simulink model "PubIfDecisionTOS_MDL"  (R2020b)
settings: configuration reference "DspaceConfig" (kept outside this file)
PostLoadFcn:
  | if any(exist('dsrtsu_mdlpostloadfcn', 'file') ~= 0), dsrtsu_mdlpostloadfcn('Execute', bdroot); end
InitFcn:
  | , if any(exist('dsmpb_private', 'file') ~= 0), dsmpb_private('dsmpb_mdlclblib', 'Init', bdroot); end,
undefined symbols (not defined in the file or in its folder): C_TOS_ACCEgoRAxletoFbumplength_m, C_TOS_ACCTargetFront_Flag, C_TOS_AEBJAPedObjDxThre_Val, C_TOS_AEBJAPedObjDyThre_Val, C_TOS_AEBJATargetSize_Val, C_TOS_AEBJAVehObjDxThre_Val, C_TOS_AEBJAVehObjDyThre_Val, C_TOS_AEBJuncPedTargetSize_Val, C_TOS_AEBLatObjDxThre_Val, C_TOS_AEBLatPedDyThre_Val, C_TOS_AEBLatTargetSize_Val, C_TOS_AEBLongTargetInEgoFront_Flag, C_TOS_axAbsGround_Parameter, C_TOS_CameraConfirmedFlag, C_TOS_CNsubjWidth, C_TOS_CurrentLaneCoreMinWidth_Val, C_TOS_CutInProb_Val_Zero, C_TOS_CutOutProb_Val_Zero, C_TOS_D2R_Val, C_TOS_DefaultValueObjectToCenterLine_dy, C_TOS_EgoCarWidth_Val, C_TOS_EgoDxRefPoint_m, C_TOS_EgoRAxletoFbumplength_m, C_TOS_HalfWidthVehicle_Con, C_TOS_HWA_CurrentLaneFlag, C_TOS_HWA_LeftLaneFlag, C_TOS_HWA_MovingDir_Vaild, C_TOS_HWA_MovState_Vaild, C_TOS_HWA_RightLaneFlag, C_TOS_LaneLineCourseErrorFront, C_TOS_LaneLineCourseErrorRear, C_TOS_MotorbikeDefaultWidth_m, C_TOS_NumberOfEffectiveTargets, C_TOS_Obj_Age_Val, C_TOS_Objdx_Constraint_Val, C_TOS_ObjectDefaultWidth_m, C_TOS_ObjInCurrentLane_Val, C_TOS_ObjInCurrentLaneValid, C_TOS_ObjInLeftLaneValid, C_TOS_ObjInRightLaneValid, C_TOS_ObjNotInCurrentLane_Val, C_TOS_ObjNotREElementType, C_TOS_ObjPredictDis_dy_ConstantVal_Zeros, C_TOS_ObjToCenterLine_ConstantVal_Zeros, C_TOS_OFMObjIDInvilad_Val, C_TOS_PIL_LatDisCons_Val_zero, C_TOS_PIL_ObjectCutInFlag_b, C_TOS_PIL_ObjectCutOutFlag_b, C_TOS_PIL_ObjLaneProb_al_Val, C_TOS_PP_ObjFusType_FC_Confirm_b, C_TOS_PP_ObjFusType_FC_FR_Confirm_b, C_TOS_PP_ObjFusType_FR_Confirm_b, C_TOS_RE_80BoolDefault_Val, C_TOS_RE_80Single181Default_Val, C_TOS_RE_80Single255Default_Val, C_TOS_RE_80Uint8Default_Val, C_TOS_RE_D2R, C_TOS_RE_D_180_Val, C_TOS_RE_InvalidObjectID_Val, C_TOS_RE_InvalidTargetChainDir_Val ... (+142)
libraries: simulink x1650, TOS_LIB x361, canfdmsglib x14
(part 5 of 69)

== system PubIfDecisionTOS_MDL/TOS_20201112/TOS_2012080320/TOS ==
  TOS_AddAttributes : Inport
  OFM_SignalVerification : Inport  Port=2
  TLJ_TargetInLaneValidityJudg : Inport  Port=3
  VIE_SignalVerification : Inport  Port=4
  PP_CenterLineCalculat : Inport  Port=5
  TOS_VCAN_SignalVerification : Inport  Port=6
  LM_SignalVerification : Inport  Port=7
  TOS_ProbInLaneCalculat : Inport  Port=8
  PP_REElementType : Inport  Port=9
  ACC : Subsystem
  AEB : Subsystem
  Bus Selector : BusSelector  OutputSignals=VIE_SignalVerification.psiDtOpt,VIE_SignalVerification.vxvRefMs
  Constant : Constant  OutDataTypeStr=boolean
  LC_LCKie_ELK : Subsystem
  OutPutPortAdaptation : Subsystem
  P0_Trajectory_V1.0 : Subsystem
  Signal Conversion{,1..12} (13 alike) : SignalConversion  OverrideOpt=off
  TOS_AEBLONOBJ : Outport  OutDataTypeStr=Bus: TOS_AEB_LONOBJ_BUS  PortDimensions=1  BusOutputAsStruct=on
  TOS_AEB_JAOBJ : Outport  Port=2  OutDataTypeStr=Bus: TOS_AEB_JAOBJ_BUS  PortDimensions=1  BusOutputAsStruct=on
  TOS_AEB_LATOBJ : Outport  Port=3  OutDataTypeStr=Bus: TOS_AEB_LATOBJ_BUS  PortDimensions=1  BusOutputAsStruct=on
  TOS_ACCP0 : Outport  Port=4  OutDataTypeStr=Bus: TOS_ACCP0_BUS  PortDimensions=1  BusOutputAsStruct=on
  TOS_ACCP1 : Outport  Port=5  OutDataTypeStr=Bus: TOS_ACCP1_BUS  PortDimensions=1  BusOutputAsStruct=on
  TOS_ACCP2 : Outport  Port=6  OutDataTypeStr=Bus: TOS_ACCP2_BUS  PortDimensions=1  BusOutputAsStruct=on
  TOS_ACCP3 : Outport  Port=7  OutDataTypeStr=Bus: TOS_ACCP3_BUS  PortDimensions=1  BusOutputAsStruct=on
  TOS_ACCP4 : Outport  Port=8  OutDataTypeStr=Bus: TOS_ACCP4_BUS  PortDimensions=1  BusOutputAsStruct=on
  TOS_ACCP5 : Outport  Port=9  OutDataTypeStr=Bus: TOS_ACCP5_BUS  PortDimensions=1  BusOutputAsStruct=on
  TOS_LC : Outport  Port=10  OutDataTypeStr=Bus: TOS_LC_BUS  PortDimensions=1  BusOutputAsStruct=on
  TOS_LCKIE : Outport  Port=11  OutDataTypeStr=Bus: TOS_LCKIE_BUS  PortDimensions=1  BusOutputAsStruct=on
  TOS_ELK : Outport  Port=12  OutDataTypeStr=Bus: TOS_ELK_BUS  PortDimensions=1  BusOutputAsStruct=on
  TEM_P0_TARGET_LINE : Outport  Port=13  OutDataTypeStr=Bus: TOS_P0_TARGET_LINE_BUS  PortDimensions=1  BusOutputAsStruct=on
  wires:
  P0_Trajectory_V1.0/1(TEM_P0_TARGET_LINE) -> Signal Conversion12/1  "TOS_TEM_P0_TARGET_LINE"
  LC_LCKie_ELK/3(TOS_ELK) -> Signal Conversion11/1  "TOS_ELK"
  LC_LCKie_ELK/2(TOS_LCKie) -> Signal Conversion10/1  "TOS_LCKIE"
  LC_LCKie_ELK/1(TOS_LC) -> Signal Conversion9/1  "TOS_LC"
  TOS_ProbInLaneCalculat/1 -> OutPutPortAdaptation/5(TOS_ProbInLaneCalculat)  "TOS_ProbInLaneCalculat"
  VIE_SignalVerification/1 -> OutPutPortAdaptation/4(VIE_SignalVerification)  "VIE_SignalVerification"
  TLJ_TargetInLaneValidityJudg/1 -> OutPutPortAdaptation/3(TLJ_TargetInLaneValidityJudg)  "TLJ_TargetInLaneValidityJudg"
  OFM_SignalVerification/1 -> OutPutPortAdaptation/2(OFM_SignalVerification)  "OFM_SignalVerification"
  TOS_AddAttributes/1 -> OutPutPortAdaptation/1(TOS_AddAttributes)  "TOS_AddAttributes"
  OutPutPortAdaptation/1(Out1) -> Bus Selector/1, LC_LCKie_ELK/1(TOSAAt_OFM_TIL_VIE), ACC/1(TOSAAt_OFM_TIL_VIE), AEB/1(TOSAAt_OFM_TIL_VIE)
  AEB/2(TOS_AEB_JAOBJ) -> Signal Conversion1/1  "TOS_AEBJuncObjInfo"
  AEB/3(TOS_AEB_LATOBJ) -> Signal Conversion2/1  "TOS_AEBLatObjInfo"
  ACC/6(TOS_ACCP5) -> Signal Conversion8/1  "TOS_ACCP5"
  ACC/5(TOS_ACCP4) -> Signal Conversion7/1  "TOS_ACCP4"
  ACC/4(TOS_ACCP3) -> Signal Conversion6/1  "TOS_ACCP3"
  ACC/3(TOS_ACCP2) -> Signal Conversion5/1  "TOS_ACCP2"
  AEB/1(TOS_AEBLONOBJ) -> Signal Conversion/1  "TOS_AEBLongObjInfo"
  ACC/2(TOS_ACCP1) -> Signal Conversion4/1  "TOS_ACCP1"
  ACC/1(TOS_ACCP0) -> Signal Conversion3/1  "TOS_ACCP0"
  PP_CenterLineCalculat/1 -> OutPutPortAdaptation/6(PP_CenterLineCalculat)  "PP_CenterLineCalculat"
  TOS_VCAN_SignalVerification/1 -> OutPutPortAdaptation/7(TOS_VCAN_SignalVerification)  "TOS_VCAN_SignalVerification"
  LM_SignalVerification/1 -> OutPutPortAdaptation/8(LM_SignalVerification)  "LM_SignalVerification"
  [TOS_ACC_P0] -> P0_Trajectory_V1.0/4(TOS_ACC_P0)
  Bus Selector/1 -> P0_Trajectory_V1.0/2(PsiDtOpt)  "<psiDtOpt>"
  Bus Selector/2 -> P0_Trajectory_V1.0/3(VxvRef_ms)  "<vxvRefMs>"
  Constant/1 -> P0_Trajectory_V1.0/1(VehStandstill)
  PP_REElementType/1 -> OutPutPortAdaptation/9(PP_REElementType)  "PP_REElementType"
  Signal Conversion/1 -> TOS_AEBLONOBJ/1
  Signal Conversion1/1 -> TOS_AEB_JAOBJ/1
  Signal Conversion2/1 -> TOS_AEB_LATOBJ/1
  Signal Conversion3/1 -> [TOS_ACC_P0], TOS_ACCP0/1
  Signal Conversion4/1 -> TOS_ACCP1/1
  Signal Conversion5/1 -> TOS_ACCP2/1
  Signal Conversion6/1 -> TOS_ACCP3/1
  Signal Conversion7/1 -> TOS_ACCP4/1
  Signal Conversion8/1 -> TOS_ACCP5/1
  Signal Conversion9/1 -> TOS_LC/1
  Signal Conversion10/1 -> TOS_LCKIE/1
  Signal Conversion11/1 -> TOS_ELK/1
  Signal Conversion12/1 -> TEM_P0_TARGET_LINE/1

== system PubIfDecisionTOS_MDL/TOS_20201112/TOS_2012080320/TOS_P0_TARGET ==
  TOS_P0_TARGET : Inport
  TOS_UpdateCnt : Inport  Port=2
  Bus Selector : BusSelector  OutputSignals=OTL_C0,OTL_C1,OTL_C2,OTL_C3,OTL_Cnt,OTL_Range,OTL_Valid
  CAN FD Pack : canfdmsglib/CAN FD Pack  CANdbFile=D:\029_HWA\05_HWA\05_详细设计文档\TOS_V3_dbc\InternalData03_ACC_AEBLog_ELK_LC_LCKie_20200927.dbc  MsgList=(none)  MsgName=TOS_P0_TARGET  ProtocolMode=CAN FD  MsgIDType=Standard (11-bit identifier)  MsgIdentifier=528  MsgLength=64  Remote=off  BRSSwitch=off  ApplyMinMax=off  SignalInfo={'{'OTL_C0','12','12','BE','unsigned','Standard','0','0.01','-16','-16','24.95';'OTL_C1','29','11','BE','unsigned','Standard','0','0.0009','-0.9','-0.9','0.9423';'OTL_C2','44','12','BE','unsigned','Standard','0','5e-06','-0.01','-0.01','0.010475';'OTL_C3','56','16','BE','unsigned','Standard','0','1e-08','-0.00033','-0.00033','0.00032535';'OTL_Cnt','64','8','BE','unsigned','Standard','0','1','0','0','255';'OTL_Range','85','11','BE','unsigned','Standard','0','0.1','0','0','204.7';'OTL_Valid','10','2','BE','unsigned','Standard','0','1','0','0','3'}
      settings: SourceProductBaseCode=VN  DataFormat=CANdb specified signals
  TOS_P0_TARGET_msg : Outport
  wires:
  CAN FD Pack/1 -> TOS_P0_TARGET_msg/1
  TOS_P0_TARGET/1 -> Bus Selector/1
  Bus Selector/1 -> CAN FD Pack/1  "<OTL_C0>"
  Bus Selector/2 -> CAN FD Pack/2  "<OTL_C1>"
  Bus Selector/3 -> CAN FD Pack/3  "<OTL_C2>"
  Bus Selector/4 -> CAN FD Pack/4  "<OTL_C3>"
  Bus Selector/5 -> CAN FD Pack/5  "<OTL_Cnt>"
  Bus Selector/6 -> CAN FD Pack/6  "<OTL_Range>"
  Bus Selector/7 -> CAN FD Pack/7  "<OTL_Valid>"
  TOS_UpdateCnt/1 -> CAN FD Pack/8

== system PubIfDecisionTOS_MDL/TOS_20201112/TOS_2012080320/PIL_1029/BoundaryCalculat ==
  OFM_SignalVerification : Inport
  TOS_AddAttributes : Inport  Port=2
  PP_Same_CenterLine : Inport  Port=3
  PP_Left_CenterLine : Inport  Port=4
  PP_Right_CenterLine : Inport  Port=5
  PP_CenterLineCalculat : Inport  Port=6
  Bus Creator1 : BusCreator  Inputs=12
  Bus Creator3 : BusCreator  Inputs=6
  Bus Creator5 : BusCreator  Inputs=3
  Bus Selector1 : BusSelector  OutputSignals=OFM_SignalVerification,TOS_AddAttributes,PP_CenterLineCalculat
  Bus Selector4 : BusSelector  OutputSignals=OFM_SignalVerification,PP_Left_CenterLine,PP_Same_CenterLine,PP_Right_CenterLine
  Lane_BoundaryCalculat : Subsystem
  ObjectToCenterLine_dyc : Subsystem
  PIL_Lane_BoundaryCalculat : Outport
  PIL_ObjectToCenterLine_dyc : Outport  Port=2
  wires:
  Lane_BoundaryCalculat/12(RightLane_BasicLaneWidth_ObserVale) -> Bus Creator1/12  "RightLane_BasicLaneWidth_ObserVale"
  Lane_BoundaryCalculat/11(LeftLane_BasicLaneWidth_ObserVale) -> Bus Creator1/11  "LeftLane_BasicLaneWidth_ObserVale"
  Lane_BoundaryCalculat/10(SameLane_BasicLaneWidth_ObserVale) -> Bus Creator1/10  "SameLane_BasicLaneWidth_ObserVale"
  Bus Creator5/1 -> PIL_ObjectToCenterLine_dyc/1  "PIL_ObjectToCenterLine_dyc"
  Lane_BoundaryCalculat/9(RightLane_EdgeRight_Boundary) -> Bus Creator1/9  "RightLane_EdgeRight_Boundary"
  Lane_BoundaryCalculat/8(RightLane_EdgeLeft_Boundary) -> Bus Creator1/8  "RightLane_EdgeLeft_Boundary"
  Lane_BoundaryCalculat/7(RightLane_CoreArea_Boundary) -> Bus Creator1/7  "RightLane_CoreArea_Boundary"
  Lane_BoundaryCalculat/6(LeftLane_EdgeRight_Boundary) -> Bus Creator1/6  "LeftLane_EdgeRight_Boundary"
  Lane_BoundaryCalculat/5(LeftLane_EdgeLeft_Boundary) -> Bus Creator1/5  "LeftLane_EdgeLeft_Boundary"
  Lane_BoundaryCalculat/4(LeftLane_CoreArea_Boundary) -> Bus Creator1/4  "LeftLane_CoreArea_Boundary"
  Lane_BoundaryCalculat/3(SameLane_EdgeRight_Boundary) -> Bus Creator1/3  "SameLane_EdgeRight_Boundary"
  Lane_BoundaryCalculat/2(SameLane_EdgeLeft_Boundary) -> Bus Creator1/2  "SameLane_EdgeLeft_Boundary"
  Lane_BoundaryCalculat/1(SameLane_CoreArea_Boundary) -> Bus Creator1/1  "SameLane_CoreArea_Boundary"
  ObjectToCenterLine_dyc/3(PIL_RightCenterLine_dyc_Filt) -> Bus Creator5/3  "PIL_RightCenterLine_dyc"
  ObjectToCenterLine_dyc/2(PIL_SameCenterLine_dyc_Filt) -> Bus Creator5/2  "PIL_SameCenterLine_dyc"
  ObjectToCenterLine_dyc/1(PIL_LeftCenterLine_dyc_Filt) -> Bus Creator5/1  "PIL_LeftCenterLine_dyc"
  Bus Selector4/1 -> ObjectToCenterLine_dyc/1(OFM_SignalVerification)  "<OFM_SignalVerification>"
  Bus Selector4/4 -> ObjectToCenterLine_dyc/4(Right_CenterLine)  "<PP_Right_CenterLine>"
  Bus Selector4/3 -> ObjectToCenterLine_dyc/3(Same_CenterLine)  "<PP_Same_CenterLine>"
  Bus Selector4/2 -> ObjectToCenterLine_dyc/2(Left_CenterLine)  "<PP_Left_CenterLine>"
  Bus Selector1/3 -> Lane_BoundaryCalculat/3(PP_CenterLineCalculat)  "<PP_CenterLineCalculat>"
  PP_CenterLineCalculat/1 -> Bus Creator3/6  "PP_CenterLineCalculat"
  Bus Creator1/1 -> PIL_Lane_BoundaryCalculat/1  "PIL_Lane_BoundaryCalculat"
  Bus Selector1/2 -> Lane_BoundaryCalculat/2(TOS_AddAttributes)  "<TOS_AddAttributes>"
  Bus Selector1/1 -> Lane_BoundaryCalculat/1(OFM_SignalVerification)  "<OFM_SignalVerification>"
  Bus Creator3/1 -> Bus Selector1/1, Bus Selector4/1
  PP_Right_CenterLine/1 -> Bus Creator3/5  "PP_Right_CenterLine"
  PP_Left_CenterLine/1 -> Bus Creator3/4  "PP_Left_CenterLine"
  PP_Same_CenterLine/1 -> Bus Creator3/3  "PP_Same_CenterLine"
  OFM_SignalVerification/1 -> Bus Creator3/1  "OFM_SignalVerification"
  TOS_AddAttributes/1 -> Bus Creator3/2  "TOS_AddAttributes"

== system PubIfDecisionTOS_MDL/TOS_20201112/TOS_2012080320/PIL_1029/ObjCutInOut_Prob ==
  PIL_ObjectToCenterLine_dy_Filt : Inport
  OFM_SignalVerification : Inport  Port=2
  TOS_AddAttributes : Inport  Port=3
  LaneWidth : Inport  Port=4
  Bus Creator : BusCreator  Inputs=4
  Bus Selector1 : BusSelector  OutputSignals=TOS_AddAttributes.PP_ObjectToCenterLine_dy,TOS_AddAttributes.PP_ObjectToCenterLine_vyc,LaneWidth.TOS_PP_CurrentLaneWidth
  Bus Selector2 : BusSelector  OutputSignals=PIL_ObjectToCenterLine_dy_Filt
  Bus Selector3 : BusSelector  OutputSignals=OFM_SignalVerification.TOS_OFMObjValid_Flag,OFM_SignalVerification.Object_Width,OFM_SignalVerification.Object_DX,OFM_SignalVerification.Object_DY,OFM_SignalVerification.Object_Age,OFM_SignalVerification.Object_Type,OFM_SignalVerification.Object_MovingState
  Bus Selector4 : BusSelector  OutputSignals=OFM_SignalVerification.TOS_OFMObjValid_Flag,OFM_SignalVerification.Object_Width,OFM_SignalVerification.Object_DX,OFM_SignalVerification.Object_DY,OFM_SignalVerification.Object_Age,OFM_SignalVerification.Object_Type,OFM_SignalVerification.Object_MovingState,OFM_SignalVerification.Object_VY,OFM_SignalVerification.Object_Std_DY
  Bus Selector5 : BusSelector  OutputSignals=TOS_AddAttributes.PP_ObjectToCenterLine_dy,TOS_AddAttributes.PP_ObjectToCenterLine_vyc
  Bus Selector6 : BusSelector  OutputSignals=PIL_ObjectToCenterLine_dy_Filt
  ObjectCutIn : Subsystem
  ObjectCutOut : Subsystem
  PIL_ObjectCutInPro_Filt : Outport
  PIL_ObjectCutIn_Flag : Outport  Port=2
  PIL_ObjectCutOutPro : Outport  Port=3
  PIL_ObjectCutOutFlag : Outport  Port=4
  wires:
  LaneWidth/1 -> Bus Creator/4  "LaneWidth"
  Bus Selector6/1 -> ObjectCutOut/12(PIL_ObjectToCenterLine_dy_Filt)  "<PIL_ObjectToCenterLine_dy_Filt>"
  Bus Selector5/2 -> ObjectCutOut/11(PP_ObjectToCenterLine_vyc)  "<PP_ObjectToCenterLine_vyc>"
  Bus Selector5/1 -> ObjectCutOut/10(PP_ObjectToCenterLine_dy)  "<PP_ObjectToCenterLine_dy>"
  Bus Selector2/1 -> ObjectCutIn/11(PIL_ObjectToCenterLine_dy_Filt)  "<PIL_ObjectToCenterLine_dy_Filt>"
  Bus Selector1/3 -> ObjectCutIn/10(PP_CurrentLaneWidth)  "<TOS_PP_CurrentLaneWidth>"
  Bus Selector1/2 -> ObjectCutIn/9(PP_ObjectToCenterLine_vyc)  "<PP_ObjectToCenterLine_vyc>"
  Bus Selector1/1 -> ObjectCutIn/8(PP_ObjectToCenterLine_dy)  "<PP_ObjectToCenterLine_dy>"
  PIL_ObjectToCenterLine_dy_Filt/1 -> Bus Creator/3  "PIL_ObjectToCenterLine_dy_Filt"
  TOS_AddAttributes/1 -> Bus Creator/2  "TOS_AddAttributes"
  OFM_SignalVerification/1 -> Bus Creator/1  "OFM_SignalVerification"
  Bus Creator/1 -> Bus Selector3/1, Bus Selector6/1, Bus Selector5/1, Bus Selector4/1, Bus Selector2/1, Bus Selector1/1
  Bus Selector4/1 -> ObjectCutOut/1(TOS_OFMObjValid_Flag)  "<TOS_OFMObjValid_Flag>"
  Bus Selector4/2 -> ObjectCutOut/2(Object_Width)  "<Object_Width>"
  Bus Selector4/3 -> ObjectCutOut/3(Object_DX)  "<Object_DX>"
  Bus Selector4/4 -> ObjectCutOut/4(Object_DY)  "<Object_DY>"
  Bus Selector4/5 -> ObjectCutOut/5(Object_Age)  "<Object_Age>"
  Bus Selector4/6 -> ObjectCutOut/6(Object_Type)  "<Object_Type>"
  Bus Selector4/7 -> ObjectCutOut/7(Object_MovingState)  "<Object_MovingState>"
  Bus Selector4/8 -> ObjectCutOut/8(Object_VY)  "<Object_VY>"
  Bus Selector4/9 -> ObjectCutOut/9(Object_Std_DY)  "<Object_Std_DY>"
  ObjectCutOut/2(TOS_PIL_ObjectCutOut_Flag) -> PIL_ObjectCutOutFlag/1
  ObjectCutOut/1(TOS_PIL_ObjectCutOutPro_Filt) -> PIL_ObjectCutOutPro/1
  Bus Selector3/1 -> ObjectCutIn/1(TOS_OFMObjValid_Flag)  "<TOS_OFMObjValid_Flag>"
  Bus Selector3/2 -> ObjectCutIn/2(Object_Width)  "<Object_Width>"
  Bus Selector3/3 -> ObjectCutIn/3(Object_DX)  "<Object_DX>"
  Bus Selector3/4 -> ObjectCutIn/4(Object_DY)  "<Object_DY>"
  Bus Selector3/5 -> ObjectCutIn/5(Object_Age)  "<Object_Age>"
  Bus Selector3/6 -> ObjectCutIn/6(Object_Type)  "<Object_Type>"
  Bus Selector3/7 -> ObjectCutIn/7(Object_MovingState)  "<Object_MovingState>"
  ObjectCutIn/1(TOS_PIL_ObjectCutInPro_Filt) -> PIL_ObjectCutInPro_Filt/1
  ObjectCutIn/2(TOS_PIL_ObjectCutIn_Flag) -> PIL_ObjectCutIn_Flag/1

== system PubIfDecisionTOS_MDL/TOS_20201112/TOS_2012080320/PIL_1029/OverlapRatio_Calculate ==
  TOS_OFMObjValid_Flag : Inport  Partition=on  PartitionDimension=1  PartitionWidth=1  PartitionOffset=0
  ObjectWidth : Inport  Port=2  Partition=on  PartitionDimension=1  PartitionWidth=1  PartitionOffset=0
  ObjectTypeCameraConfirmed : Inport  Port=3  Partition=on  PartitionDimension=1  PartitionWidth=1  PartitionOffset=0
  object_MovingState : Inport  Port=4  Partition=on  PartitionDimension=1  PartitionWidth=1  PartitionOffset=0
  Object_Type : Inport  Port=5  Partition=on  PartitionDimension=1  PartitionWidth=1  PartitionOffset=0
  dyEgo2Center : Inport  Port=6
  dyObject2Center : Inport  Port=7  Partition=on  PartitionDimension=1  PartitionWidth=1  PartitionOffset=0
  Compare To Constant : simulink/Logic and Bit Operations/Compare To Constant  relop===  const=C_TOS_OFMObjIDInvilad_Val  OutDataTypeStr=boolean
      settings: AttributesFormatString=C_TOS_OFMObjIDInvilad_Val = 0
  For Each : ForEach  DisableCoverage=on
  If : If  IfExpression=u1 ~= 0
  Merge : Merge
  OverlapCalculation_Default : Subsystem  TreatAsAtomicUnit=on
  PIL_OverlapCalculation : Subsystem  TreatAsAtomicUnit=on
  PIL_OverlapRatio : Outport  OutDataTypeStr=single  ConcatenationDimension=1
  wires:
  dyObject2Center/1 -> PIL_OverlapCalculation/6(dyObject2Center)
  dyEgo2Center/1 -> PIL_OverlapCalculation/5(dyEgo2Center)
  object_MovingState/1 -> PIL_OverlapCalculation/3(object_MovingState)
  ObjectTypeCameraConfirmed/1 -> PIL_OverlapCalculation/2(ObjectTypeCameraConfirmed)
  ObjectWidth/1 -> PIL_OverlapCalculation/1(ObjectWidth)
  OverlapCalculation_Default/1(PIL_overlapRatio) -> Merge/1
  Merge/1 -> PIL_OverlapRatio/1
  If/1 -> OverlapCalculation_Default/Action
  Compare To Constant/1 -> If/1
  TOS_OFMObjValid_Flag/1 -> Compare To Constant/1
  PIL_OverlapCalculation/1(overlapRatio) -> Merge/2
  If/2 -> PIL_OverlapCalculation/Action
  Object_Type/1 -> PIL_OverlapCalculation/4(Object_Type)

== system PubIfDecisionTOS_MDL/TOS_20201112/TOS_2012080320/PIL_1029/PIL_ObjectToCenterLine_dy_Filt ==
  note: fun: 目标到本车道中心线距离滤波
  ObjectToCenterLine_dy : Inport
  TOS_OFMObjValid_Flag : Inport  Port=2
  Object_ID : Inport  Port=3  OutDataTypeStr=uint8
  Object_Age : Inport  Port=4
  PIL_ObjectToCenterLine_dy : Subsystem
  Unit Delay : UnitDelay  InitialCondition=zeros(80,1)  SampleTime=-1  HasFrameUpgradeWarning=on
      settings: AttributesFormatString=initVal = zeros(80,1)
  Unit Delay1 : UnitDelay  InitialCondition=ones(80,1)*255  SampleTime=-1  HasFrameUpgradeWarning=on
      settings: AttributesFormatString=initVal = ones(80,1)*255
  PIL_ObjectToCenterLine_dy_Filt : Outport  OutDataTypeStr=single
  wires:
  TOS_OFMObjValid_Flag/1 -> PIL_ObjectToCenterLine_dy/4(TOS_OFMObjValid_Flag)
  Object_Age/1 -> PIL_ObjectToCenterLine_dy/6(Object_Age)
  ObjectToCenterLine_dy/1 -> PIL_ObjectToCenterLine_dy/3(ObjectToCenterLine_dy)
  PIL_ObjectToCenterLine_dy/2(ObjectToCenterLine_dy_Filt) -> PIL_ObjectToCenterLine_dy_Filt/1, Unit Delay1/1  "TOS_PIL_ObjectToCenterLine_dy_Filt"
  Unit Delay1/1 -> PIL_ObjectToCenterLine_dy/2(ObjectToCenterLine_dy_Filt_K1)
  Object_ID/1 -> PIL_ObjectToCenterLine_dy/5(Object_ID)
  PIL_ObjectToCenterLine_dy/1(Obj_ID) -> Unit Delay/1
  Unit Delay/1 -> PIL_ObjectToCenterLine_dy/1(ObjectID_Filt_K1)

== system PubIfDecisionTOS_MDL/TOS_20201112/TOS_2012080320/PIL_1029/ProbCalculat ==
  CurrentLane_LeftRightLine : Inport
  OFM_SignalVerification : Inport  Port=2
  TOS_AddAttributes : Inport  Port=3
  LM_SignalVerification : Inport  Port=4
  PIL_Lane_BoundaryCalculat : Inport  Port=5
  PIL_ObjectToCenterLine_dyc : Inport  Port=6
  Bus Creator : BusCreator  Inputs=6
  Bus Selector : BusSelector  OutputSignals=OFM_SignalVerification,PIL_Lane_BoundaryCalculat,PIL_ObjectToCenterLine_dyc,LM_SignalVerification
  ProbCalculat : Subsystem
  ProbFilt : Subsystem
  PIL_ObjinEgoLaneProb_Filt : Outport  OutDataTypeStr=single
  PIL_ObjinLeftLaneProb_Filt : Outport  Port=2  OutDataTypeStr=single
  PIL_ObjinRightLaneProb_Filt : Outport  Port=3  OutDataTypeStr=single
  "PIL_ObjLaneProb_all " : Outport  Port=4
  PIL_EgoVehicleProFilt : Outport  Port=5
  wires:
  ProbFilt/1(PIL_ObjinEgoLaneProb_Filt) -> [TOS_PIL_SameLanePro_Filt], PIL_ObjinEgoLaneProb_Filt/1
  ProbFilt/3(PIL_ObjinRightLaneProb_Filt) -> [PIL_RightLaneProb_Filt], PIL_ObjinRightLaneProb_Filt/1
  ProbFilt/2(PIL_ObjinLeftLaneProb_Filt) -> [PIL_LeftLaneProb_Filt], PIL_ObjinLeftLaneProb_Filt/1
  Bus Creator/1 -> [OFM_InPutSig], Bus Selector/1
  ProbCalculat/3(PIL_RightLaneProb) -> ProbFilt/4(PIL_ObjinRightLaneProb), [TOS_PIL_RightLaneProb]
  ProbCalculat/2(PIL_LeftLaneProb) -> ProbFilt/3(PIL_ObjinLeftLaneProb), [PIL_LeftLaneProb]
  Bus Selector/3 -> ProbCalculat/3(PIL_ObjectToCenterLine_dyc)  "<PIL_ObjectToCenterLine_dyc>"
  TOS_AddAttributes/1 -> Bus Creator/3  "TOS_AddAttributes"
  CurrentLane_LeftRightLine/1 -> Bus Creator/1  "CurrentLane_LeftRightLine"
  Bus Selector/2 -> ProbCalculat/2(CurrentLane_Boundary)  "<PIL_Lane_BoundaryCalculat>"
  Bus Selector/1 -> ProbCalculat/1(OFM_SignalVerification)  "<OFM_SignalVerification>"
  PIL_ObjectToCenterLine_dyc/1 -> Bus Creator/6  "PIL_ObjectToCenterLine_dyc"
  PIL_Lane_BoundaryCalculat/1 -> Bus Creator/5  "PIL_Lane_BoundaryCalculat"
  OFM_SignalVerification/1 -> Bus Creator/2  "OFM_SignalVerification"
  ProbCalculat/1(PIL_EgoLaneProb) -> ProbFilt/2(PIL_ObjinEgoLaneProb), [PIL_CurrentLaneProb]
  LM_SignalVerification/1 -> Bus Creator/4  "LM_SignalVerification"
  Bus Selector/4 -> ProbCalculat/4(LM_SignalVerification)  "<LM_SignalVerification>"
  ProbCalculat/5(PIL_EgoVehicleProFilt) -> [PIL_EgoVehicleProFilt], PIL_EgoVehicleProFilt/1
  ProbCalculat/4("PIL_ObjLaneProb_all ") -> "PIL_ObjLaneProb_all "/1
  [OFM_InPutSig] -> ProbFilt/1(OFM_InPutSig)

== system PubIfDecisionTOS_MDL/TOS_20201112/TOS_2012080320/PP1128/AAT-AdditionalAttributes ==
  LM_SignalVerification : Inport
  OFM_Info : Inport  Port=2
  VIE_SignalVerification : Inport  Port=3
  Bus Creator : BusCreator  Inputs=3
  Bus Creator1 : BusCreator  Inputs=14  OutDataTypeStr=Bus: TOS_AddAttributes_BUS  NonVirtualBus=on
      settings: InheritFromInputs=off
  Bus Creator3 : BusCreator  Inputs=4
  Bus Selector : BusSelector  OutputSignals=OFM_SignalVerification.Object_MovingState,OFM_SignalVerification.Object_Orientation,OFM_SignalVerification.Object_AX,VIE_SignalVerification.axvRefMs2,OFM_SignalVerification.Object_MovingState,OFM_SignalVerification.Object_Fus_Type,OFM_SignalVerification.Object_DX,OFM_SignalVerification.TOS_OFMObjValid_Flag
  Bus Selector1 : BusSelector  OutputSignals=OFM_SignalVerification,LM_SignalVerification,VIE_SignalVerification
  Bus Selector3 : BusSelector  OutputSignals=OFM_SignalVerification.Object_DX,OFM_SignalVerification.Object_DY,OFM_SignalVerification.Object_ID,OFM_SignalVerification.TOS_OFMObjValid_Flag
  Bus Selector5 : BusSelector  OutputSignals=OFM_SignalVerification,LM_SignalVerification,VIE_SignalVerification.vxvRefMs
  Bus Selector6 : BusSelector  OutputSignals=OFM_SignalVerification,LM_SignalVerification
  PP_CenterLine_Calculat : Subsystem
  PP_ObjFirstDxDyDetermineSignalProcessing : Subsystem
  PP_ObjectToCenterLine_dy : Subsystem
  PP_SignalProcessing : Subsystem
  RoadEdge : Subsystem
  TAP_TargetPreprocessing : Subsystem
  TOS_AddAttributes : Outport
  PP_CenterLineCalculat : Outport  Port=2
  OFM_SignalVerification : Outport  Port=3
  PP_REElementType : Outport  Port=4
  wires:
  LM_SignalVerification/1 -> Bus Creator/3  "LM_SignalVerification"
  OFM_Info/1 -> TAP_TargetPreprocessing/1(OFM_Info)  "OFM_SignalVerification"
  Bus Selector5/1 -> PP_ObjectToCenterLine_dy/1("OFM_SignalVerification ")  "<OFM_SignalVerification>"
  Bus Selector5/2 -> PP_ObjectToCenterLine_dy/2(LM_SignalVerification)  "<LM_SignalVerification>"
  PP_ObjectToCenterLine_dy/2(PP_ObjectToCenterLine_dy) -> Bus Creator1/11  "TOS_PP_ObjectToCenterLine_dy"
  VIE_SignalVerification/1 -> Bus Creator/2  "VIE_SignalVerification"
  Bus Creator1/1 -> TOS_AddAttributes/1  "TOS_PP_AddAttributes_bus"
  Bus Selector3/1 -> PP_ObjFirstDxDyDetermineSignalProcessing/1(Object_DX)  "<Object_DX>"
  Bus Selector3/2 -> PP_ObjFirstDxDyDetermineSignalProcessing/2(Object_DY)  "<Object_DY>"
  Bus Selector3/3 -> PP_ObjFirstDxDyDetermineSignalProcessing/3(Object_ID)  "<Object_ID>"
  PP_ObjectToCenterLine_dy/1(PP_EgoVehCenterLine_dy) -> Bus Creator1/10  "TOS_PP_EgoVehCenterLine_dy"
  PP_ObjFirstDxDyDetermineSignalProcessing/1(PP_ObjFirstDetect_Dx) -> Bus Creator1/13  "PP_ObjFirstDetect_Dx"
  PP_ObjFirstDxDyDetermineSignalProcessing/2(PP_ObjFirstDetect_Dy) -> Bus Creator1/14  "PP_ObjFirstDetect_Dy"
  PP_ObjectToCenterLine_dy/3(PP_ObjectToCenterLine_Vyc) -> Bus Creator1/12  "PP_ObjectToCenterLine_vyc"
  Bus Selector5/3 -> PP_ObjectToCenterLine_dy/3(vxvRefMs)  "<vxvRefMs>"
  Bus Selector/1 -> PP_SignalProcessing/1(Object_MovingState)  "<Object_MovingState>"
  Bus Selector/2 -> PP_SignalProcessing/2(Object_Orientation)  "<Object_Orientation>"
  Bus Selector/3 -> PP_SignalProcessing/3(Object_AX)  "<Object_AX>"
  Bus Selector/4 -> PP_SignalProcessing/4(axvRefMs2)  "<axvRefMs2>"
  Bus Selector/5 -> PP_SignalProcessing/5(Object_MovingState1)  "<Object_MovingState>"
  Bus Selector/6 -> PP_SignalProcessing/6(Object_Fus_Type)  "<Object_Fus_Type>"
  Bus Selector/7 -> PP_SignalProcessing/7(Object_DX)  "<Object_DX>"
  PP_SignalProcessing/1(PP_MovingStateSignalProcessing) -> Bus Creator1/1  "PP_MovingStateSignalProcessing"
  PP_SignalProcessing/4(PP_axAbsGround) -> Bus Creator1/4  "PP_axAbsGround"
  PP_SignalProcessing/5(PP_CamareConfirmSignalProcessing) -> Bus Creator1/5  "PP_CamareConfirmSignalProcessing"
  PP_SignalProcessing/6(PP_ObjToEgoCarFrontbump) -> Bus Creator1/6  "PP_ObjToEgoCarFrontbump"
  PP_CenterLine_Calculat/4(PP_LaneWidth) -> Bus Creator3/4
  Bus Creator3/1 -> PP_CenterLineCalculat/1  "PP_CenterLineCalculat"
  PP_CenterLine_Calculat/3(PP_RightLane_CenterLine) -> Bus Creator3/3
  PP_CenterLine_Calculat/2(PP_LeftLane_CenterLine) -> Bus Creator3/2
  Bus Selector6/2 -> PP_CenterLine_Calculat/2(LM_SignalVerification)  "<LM_SignalVerification>"
  PP_CenterLine_Calculat/1(PP_EgoLane_CenterLine) -> Bus Creator3/1
  Bus Selector/8 -> PP_SignalProcessing/8(TOS_OFMObjValid_Flag)  "<TOS_OFMObjValid_Flag>"
  PP_SignalProcessing/3(PP_ObjMovingDirSignalProcessing) -> Bus Creator1/3  "PP_ObjMovingDirSignalProcessing"
  TAP_TargetPreprocessing/1(OFM_SignalVerification) -> OFM_SignalVerification/1, Bus Creator/1  "OFM_SignalVerification"
  Bus Selector3/4 -> PP_ObjFirstDxDyDetermineSignalProcessing/4(TOS_OFMObjValid_Flag)  "<TOS_OFMObjValid_Flag>"
  PP_SignalProcessing/7(PP_ObjFusType_FC_FR_Confirm) -> Bus Creator1/7  "PP_ObjFusType_FC_FR_Confirm"
  PP_SignalProcessing/8(PP_ObjFusType_FR_Confirm) -> Bus Creator1/8  "PP_ObjFusType_FR_Confirm"
  PP_SignalProcessing/9(PP_ObjFusType_FC_Confirm) -> Bus Creator1/9  "PP_ObjFusType_FC_Confirm"
  Bus Selector6/1 -> PP_CenterLine_Calculat/1(OFM_SignalVerification)  "<OFM_SignalVerification>"
  PP_SignalProcessing/2(PP_MovingState_AEB_SignalProcessing) -> Bus Creator1/2  "PP_MovingState_AEB_SignalProcessing"
  Bus Selector1/3 -> RoadEdge/3(VIE_SignalVerification)  "<VIE_SignalVerification>"
  Bus Selector1/1 -> RoadEdge/1(OFM_SignalVerification)  "<OFM_SignalVerification>"
  RoadEdge/1(RE_EdgeElementType) -> PP_REElementType/1
  Bus Selector1/2 -> RoadEdge/2(LM_SignalVerification)  "<LM_SignalVerification>"
  Bus Creator/1 -> Bus Selector/1, Bus Selector1/1, Bus Selector6/1, Bus Selector3/1, Bus Selector5/1

== system PubIfDecisionTOS_MDL/TOS_20201112/TOS_2012080320/PP1128/ISV_InputSignalVerification ==
  OFMInfo : Inport
  vxvRefMs : Inport  Port=2
  psiDtOpt : Inport  Port=3  Interpolate=off
  kapTraj : Inport  Port=4
  axvRefMs2 : Inport  Port=5
  TOS_VCAN_CSA : Inport  Port=6  BusOutputAsStruct=on
  LM_LINE_LL : Inport  Port=7  BusOutputAsStruct=on
  LM_LINE_LR : Inport  Port=8  BusOutputAsStruct=on
  LM_LINE_RL : Inport  Port=9  BusOutputAsStruct=on
  LM_LINE_RR : Inport  Port=10  BusOutputAsStruct=on
  LM_SpecialRoadType : Inport  Port=11  OutDataTypeStr=uint8  PortDimensions=1  BusOutputAsStruct=on
  LM_RoadNumChgType : Inport  Port=12  OutDataTypeStr=uint8  PortDimensions=1  BusOutputAsStruct=on
  LM_DrivInWLType : Inport  Port=13  OutDataTypeStr=uint8  PortDimensions=1  BusOutputAsStruct=on
  LM_SignalVerif : Subsystem
  OFM_SignalVerif : Subsystem
  VIE_SignalVerif : Subsystem
  LM_SignalVerification : Outport
  OFM_SignalVerification : Outport  Port=2
  VIE_SignalVerification : Outport  Port=3
  TOS_VCAN_SignalVerification : Outport  Port=4
  wires:
  TOS_VCAN_CSA/1 -> TOS_VCAN_SignalVerification/1
  OFMInfo/1 -> OFM_SignalVerif/1(OFMInfo)  "OFMInfo"
  OFM_SignalVerif/1(OFM_SignalVerification) -> OFM_SignalVerification/1
  vxvRefMs/1 -> VIE_SignalVerif/1(vxvRefMs)
  psiDtOpt/1 -> VIE_SignalVerif/2(psiDtOpt)
  kapTraj/1 -> VIE_SignalVerif/3(kapTraj)
  axvRefMs2/1 -> VIE_SignalVerif/4(axvRefMs2)
  VIE_SignalVerif/1(VIE_SignalVerification) -> VIE_SignalVerification/1
  LM_LINE_LL/1 -> LM_SignalVerif/1(LM_LINE_LL)
  LM_LINE_LR/1 -> LM_SignalVerif/2(LM_LINE_LR)
  LM_LINE_RL/1 -> LM_SignalVerif/3(LM_LINE_RL)
  LM_LINE_RR/1 -> LM_SignalVerif/4(LM_LINE_RR)
  LM_SpecialRoadType/1 -> LM_SignalVerif/5(LM_SpecialRoadType)
  LM_RoadNumChgType/1 -> LM_SignalVerif/6(LM_RoadNumChgType)
  LM_DrivInWLType/1 -> LM_SignalVerif/7(LM_DrivInWLType)
  LM_SignalVerif/1(LM_SignalVerification) -> LM_SignalVerification/1

== system PubIfDecisionTOS_MDL/TOS_20201112/TOS_2012080320/Subsystem/For Each Subsystem ==
  In1 : Inport  Partition=on  PartitionDimension=1  PartitionWidth=1  PartitionOffset=0
  Bus Selector2 : BusSelector  OutputSignals=FusionType,ObjectID,ObjectMovingOrientation,ObjectMovingState,ObjectType,dx,dy
  For Each : ForEach  DisableCoverage=on
  FusionType : Outport  ConcatenationDimension=1
  ObjectID : Outport  Port=2  ConcatenationDimension=1
  ObjectMovingOrientation : Outport  Port=3  ConcatenationDimension=1
  ObjectMovingState : Outport  Port=4  ConcatenationDimension=1
  ObjectType : Outport  Port=5  ConcatenationDimension=1
  dx : Outport  Port=6  ConcatenationDimension=1
  dy : Outport  Port=7  ConcatenationDimension=1
  wires:
  In1/1 -> Bus Selector2/1
  Bus Selector2/1 -> FusionType/1  "<FusionType>"
  Bus Selector2/2 -> ObjectID/1  "<ObjectID>"
  Bus Selector2/3 -> ObjectMovingOrientation/1  "<ObjectMovingOrientation>"
  Bus Selector2/4 -> ObjectMovingState/1  "<ObjectMovingState>"
  Bus Selector2/5 -> ObjectType/1  "<ObjectType>"
  Bus Selector2/6 -> dx/1  "<dx>"
  Bus Selector2/7 -> dy/1  "<dy>"

== system PubIfDecisionTOS_MDL/TOS_20201112/TOS_2012080320/Subsystem/For Each Subsystem1 ==
  In1 : Inport  Partition=on  PartitionDimension=1  PartitionWidth=1  PartitionOffset=0
  Bus Selector2 : BusSelector  OutputSignals=FusionType,ObjectID,ObjectMovingOrientation,ObjectMovingState,ObjectType,dx,dy
  For Each : ForEach  DisableCoverage=on
  FusionType : Outport  ConcatenationDimension=1
  ObjectID : Outport  Port=2  ConcatenationDimension=1
  ObjectMovingOrientation : Outport  Port=3  ConcatenationDimension=1
  ObjectMovingState : Outport  Port=4  ConcatenationDimension=1
  ObjectType : Outport  Port=5  ConcatenationDimension=1
  dx : Outport  Port=6  ConcatenationDimension=1
  dy : Outport  Port=7  ConcatenationDimension=1
  wires:
  Bus Selector2/7 -> dy/1  "<dy>"
  Bus Selector2/6 -> dx/1  "<dx>"
  Bus Selector2/5 -> ObjectType/1  "<ObjectType>"
  Bus Selector2/4 -> ObjectMovingState/1  "<ObjectMovingState>"
  Bus Selector2/3 -> ObjectMovingOrientation/1  "<ObjectMovingOrientation>"
  Bus Selector2/2 -> ObjectID/1  "<ObjectID>"
  Bus Selector2/1 -> FusionType/1  "<FusionType>"
  In1/1 -> Bus Selector2/1

== system PubIfDecisionTOS_MDL/TOS_20201112/TOS_2012080320/TLJ/Pro ==
  TOS_OFMObjValid_Flag : Inport  Partition=on  PartitionDimension=1  PartitionWidth=1  PartitionOffset=0
  PIL_ObjLaneProb_all : Inport  Port=2  Partition=on  PartitionDimension=1  PartitionWidth=1  PartitionOffset=0
  PIL_EgoLaneProb : Inport  Port=3  Partition=on  PartitionDimension=1  PartitionWidth=1  PartitionOffset=0
  PIL_LeftLaneProb : Inport  Port=4  Partition=on  PartitionDimension=1  PartitionWidth=1  PartitionOffset=0
  PIL_RightLaneProb : Inport  Port=5  Partition=on  PartitionDimension=1  PartitionWidth=1  PartitionOffset=0
  PIL_EgoVehicle_EgoLaneProb : Inport  Port=6
  PIL_EgoVehicle_LeftLaneProb : Inport  Port=7
  PIL_EgoVehicle_RightLaneProb : Inport  Port=8
  Object_Type : Inport  Port=9  Partition=on  PartitionDimension=1  PartitionWidth=1  PartitionOffset=0
  Object_DY : Inport  Port=10  Partition=on  PartitionDimension=1  PartitionWidth=1  PartitionOffset=0
  PIL_CutinFlag : Inport  Port=11  Partition=on  PartitionDimension=1  PartitionWidth=1  PartitionOffset=0
  PIL_CutoutFlag : Inport  Port=12  Partition=on  PartitionDimension=1  PartitionWidth=1  PartitionOffset=0
  Compare To Constant : simulink/Logic and Bit Operations/Compare To Constant  relop=~=  const=C_TOS_OFMObjIDInvilad_Val  OutDataTypeStr=boolean
      settings: AttributesFormatString=C_TOS_OFMObjIDInvilad_Val = 0
  Compare To Constant1 : simulink/Logic and Bit Operations/Compare To Constant  relop=>=  const=C_TOS_PIL_ObjLaneProb_al_Val  OutDataTypeStr=boolean
      settings: AttributesFormatString=C_TOS_PIL_ObjLaneProb_al_Val = 0.2
  For Each : ForEach  DisableCoverage=on
  If : If  IfExpression=u1 == 0
  Logical Operator2 : Logic  AllPortsSameDT=off  OutDataTypeStr=boolean
  Merge{1..7} (7 alike) : Merge
  ObjInLane_Default : Subsystem  TreatAsAtomicUnit=on
  Pro : Subsystem
  TLJ_ObjInLeftLane_flag : Outport  ConcatenationDimension=1
  TLJ_ObjInEgoLane_flag : Outport  Port=2  ConcatenationDimension=1
  TLJ_ObjInRightLane_flag : Outport  Port=3  ConcatenationDimension=1
  TOS_TLJ_ObjinLeftLaneProb_ObserVale : Outport  Port=4  ConcatenationDimension=1
  TOS_TLJ_ObjinEgoLaneProb_ObserVale : Outport  Port=5  ConcatenationDimension=1
  TOS_TLJ_ObjinRightLaneProb_ObserVale : Outport  Port=6  ConcatenationDimension=1
  TOS_TLJ_ObjInLaneCondition_Flag_ObserVale : Outport  Port=7  ConcatenationDimension=1
  wires:
  TOS_OFMObjValid_Flag/1 -> Compare To Constant/1
  Compare To Constant/1 -> Logical Operator2/1
  PIL_ObjLaneProb_all/1 -> Compare To Constant1/1
  PIL_EgoLaneProb/1 -> Pro/1(PIL_EgoLaneProb)  "PIL_EgoLaneProb"
  PIL_LeftLaneProb/1 -> Pro/2(PIL_LeftLaneProb)  "PIL_LeftLaneProb"
  PIL_RightLaneProb/1 -> Pro/3(PIL_RightLaneProb)  "PIL_RightLaneProb"
  PIL_EgoVehicle_LeftLaneProb/1 -> Pro/5(PIL_EgoVehicle_LeftLaneProb)  "PIL_EgoVehicle_LeftLaneProb"
  PIL_EgoVehicle_EgoLaneProb/1 -> Pro/4(PIL_EgoVehicle_EgoLaneProb)  "PIL_EgoVehicle_EgoLaneProb"
  PIL_EgoVehicle_RightLaneProb/1 -> Pro/6(PIL_EgoVehicle_RightLaneProb)  "PIL_EgoVehicle_RightLaneProb"
  Compare To Constant1/1 -> Logical Operator2/2
  Logical Operator2/1 -> If/1
  If/2 -> Pro/Action
  If/1 -> ObjInLane_Default/Action
  PIL_CutinFlag/1 -> Pro/9(PIL_CutinFlag)  "PIL_CutinFlag"
  Object_Type/1 -> Pro/7(Object_Type)  "Object_Type"
  Merge3/1 -> TLJ_ObjInRightLane_flag/1
  Merge2/1 -> TLJ_ObjInEgoLane_flag/1
  ObjInLane_Default/3(TLJ_ObjInRightLane_flag) -> Merge3/1
  Pro/2(TLJ_ObjInEgoLane_flag) -> Merge2/2
  ObjInLane_Default/1(TLJ_ObjInLeftLane_flag) -> Merge1/1
  Merge1/1 -> TLJ_ObjInLeftLane_flag/1
  ObjInLane_Default/2(TLJ_ObjInEgoLane_flag) -> Merge2/1
  Pro/1(TLJ_ObjInLeftLane_flag) -> Merge1/2
  Pro/3(TLJ_ObjInRightLane_flag) -> Merge3/2
  Pro/4(TOS_TLJ_ObjinLeftLaneProb_ObserVale) -> Merge4/2
  Pro/5(TOS_TLJ_ObjinEgoLaneProb_ObserVale) -> Merge5/2
  Pro/6(TOS_TLJ_ObjinRightLaneProb_ObserVale) -> Merge6/2
  Pro/7(TOS_TLJ_ObjInLaneCondition_Flag_ObserVale) -> Merge7/2
  ObjInLane_Default/4(TOS_TLJ_ObjinLeftLaneProb_ObserVale) -> Merge4/1
  ObjInLane_Default/5(TOS_TLJ_ObjinEgoLaneProb_ObserVale) -> Merge5/1
  ObjInLane_Default/6(TOS_TLJ_ObjinRightLaneProb_ObserVale) -> Merge6/1
  ObjInLane_Default/7(TOS_TLJ_ObjInLaneCondition_Flag_ObserVale) -> Merge7/1
  Merge4/1 -> TOS_TLJ_ObjinLeftLaneProb_ObserVale/1
  Merge5/1 -> TOS_TLJ_ObjinEgoLaneProb_ObserVale/1
  Merge6/1 -> TOS_TLJ_ObjinRightLaneProb_ObserVale/1
  Merge7/1 -> TOS_TLJ_ObjInLaneCondition_Flag_ObserVale/1
  Object_DY/1 -> Pro/8(Object_DY)  "Object_DY"
  PIL_CutoutFlag/1 -> Pro/10(PIL_CutoutFlag)  "PIL_CutinFlag"

== system PubIfDecisionTOS_MDL/TOS_20201112/TOS_2012080320/TOS/ACC ==
  TOSAAt_OFM_TIL_VIE : Inport
  TOS_ACCCurrentLane : Subsystem
  TOS_ACCLeftLane : Subsystem
  TOS_ACCRightLane : Subsystem
  TOS_ACCP0 : Outport
  TOS_ACCP1 : Outport  Port=2
  TOS_ACCP2 : Outport  Port=3
  TOS_ACCP3 : Outport  Port=4
  TOS_ACCP4 : Outport  Port=5
  TOS_ACCP5 : Outport  Port=6
  wires:
  TOS_ACCRightLane/1(TOS_ACCP3) -> TOS_ACCP3/1
  TOS_ACCRightLane/2(TOS_ACCP5) -> TOS_ACCP5/1
  TOS_ACCLeftLane/2(TOS_ACCPO4) -> TOS_ACCP4/1
  TOS_ACCLeftLane/1(TOS_ACCPO2) -> TOS_ACCP2/1
  TOS_ACCCurrentLane/2(TOS_ACCP1) -> TOS_ACCP1/1
  TOS_ACCCurrentLane/1(TOS_ACCP0) -> TOS_ACCP0/1
  TOSAAt_OFM_TIL_VIE/1 -> TOS_ACCCurrentLane/1(TOSAAt_OFM_TIL_VIE), TOS_ACCLeftLane/1(TOSAAt_OFM_TIL_VIE), TOS_ACCRightLane/1(TOSAAt_OFM_TIL_VIE)

== system PubIfDecisionTOS_MDL/TOS_20201112/TOS_2012080320/TOS/AEB ==
  TOSAAt_OFM_TIL_VIE : Inport
  TOS_AEBJunct1105 : Subsystem  Commented=on
  TOS_AEBJunct_20201208 : Subsystem
  TOS_AEBLatCro1105 : Subsystem  Commented=on
  TOS_AEBLatCro_20201208 : Subsystem
  TOS_AEBLong : Subsystem
  TOS_AEBLONOBJ : Outport
  TOS_AEB_JAOBJ : Outport  Port=2
  TOS_AEB_LATOBJ : Outport  Port=3
  wires:
  TOS_AEBLatCro_20201208/1(TOS_AEB_LATOBJ) -> TOS_AEB_LATOBJ/1
  TOSAAt_OFM_TIL_VIE/1 -> TOS_AEBLatCro_20201208/1(TOSAAt_OFM_TIL_VIE), TOS_AEBJunct_20201208/1(TOSAAt_OFM_TIL_VIE), TOS_AEBLong/1(TOSAAt_OFM_TIL_VIE)
  TOS_AEBLong/1(TOS_AEBLONOBJ) -> TOS_AEBLONOBJ/1
  TOS_AEBJunct_20201208/1(TOS_AEB_JAOBJ) -> TOS_AEB_JAOBJ/1

== system PubIfDecisionTOS_MDL/TOS_20201112/TOS_2012080320/TOS/LC_LCKie_ELK ==
  TOSAAt_OFM_TIL_VIE : Inport
  ELK_TargetInfor : Subsystem
  HWA_TargetInfor : Subsystem
  LCKie_TargetInfor : Subsystem
  TOS_HWA : Subsystem
  Vector Concatenate : Concatenate  NumInputs=11  ConcatenateDimension=11
  TOS_LC : Outport
  TOS_LCKie : Outport  Port=2
  TOS_ELK : Outport  Port=3
  wires:
  [HWA_ObjectIn_Lane_b] -> HWA_TargetInfor/3(ObjectIn_Lane_b)
  TOS_HWA/12(ObjectIn_Lane_b) -> [HWA_ObjectIn_Lane_b]
  TOS_HWA/8(HWA_RightRear_Target_4) -> Vector Concatenate/8  "HWA_RighRear_Target_4"
  TOS_HWA/7(HWA_RightRear_Target_3) -> Vector Concatenate/7  "HWA_RightRear_Target_3"
  TOS_HWA/2(HWA_LeftFront_Target_2) -> Vector Concatenate/2  "HWA_LeftFront_Target2"
  TOS_HWA/3(HWA_LeftRear_Target_3) -> Vector Concatenate/3  "HWA_LeftRear_Target3"
  TOS_HWA/4(HWA_LeftRear_Target_4) -> Vector Concatenate/4  "HWA_LeftRear_Target4"
  TOS_HWA/6(HWA_RightFront_Target_2) -> Vector Concatenate/6  "HWA_RightFront_Target_2"
  TOS_HWA/1(HWA_LeftFront_Target_1) -> Vector Concatenate/1  "HWA_LeftFront_Target1"
  TOS_HWA/5(HWA_RightFront_Target_1) -> Vector Concatenate/5  "HWA_RightFront_Target_1"
  TOS_HWA/9(HWA_CurrentFront_Target_1) -> Vector Concatenate/9  "HWA_CurrentFront_Target1"
  TOS_HWA/10(HWA_CurrentFront_Target_2) -> Vector Concatenate/10  "HWA_CurrentFront_Target2"
  TOS_HWA/11(HWA_CurrentRear_Target_3) -> Vector Concatenate/11  "HWA_CurrenRear_Target1"
  HWA_TargetInfor/1(TOS_HWA_Target) -> [TOS_HWA_CurrentFront_Target_2], TOS_LC/1
  [TOSAAt_OFM_TIL_VIE] -> HWA_TargetInfor/2(TOSAAt_OFM_TIL_VIE)
  [TOSAAt_OFM_TIL_VIE] -> LCKie_TargetInfor/2(TOSAAt_OFM_TIL_VIE)
  [HWA_ObjectIn_Lane_b] -> LCKie_TargetInfor/3(ObjectIn_Lane_b)
  LCKie_TargetInfor/1(TOS_LCKIETarget) -> TOS_LCKie/1
  ELK_TargetInfor/1(TOS_ELKTarget) -> TOS_ELK/1
  [HWA_ObjectIn_Lane_b] -> ELK_TargetInfor/3(ObjectIn_Lane_b)
  Vector Concatenate/1 -> ELK_TargetInfor/1(TOS_HWA_TargetIndexVector), LCKie_TargetInfor/1(TOS_HWA_TargetIndexVector), HWA_TargetInfor/1(TOS_HWA_TargetIndexVector)
  [TOSAAt_OFM_TIL_VIE] -> ELK_TargetInfor/2(TOSAAt_OFM_TIL_VIE)
  TOSAAt_OFM_TIL_VIE/1 -> TOS_HWA/1(TOSAAt_OFM_TIL_VIE), [TOSAAt_OFM_TIL_VIE]
  [TOS_HWA_CurrentFront_Target_2] -> TOS_HWA/2(TOS_HWA_CurrentFront_Target_2)

== system PubIfDecisionTOS_MDL/TOS_20201112/TOS_2012080320/TOS/OutPutPortAdaptation ==
  TOS_AddAttributes : Inport
  OFM_SignalVerification : Inport  Port=2
  TLJ_TargetInLaneValidityJudg : Inport  Port=3
  VIE_SignalVerification : Inport  Port=4
  TOS_ProbInLaneCalculat : Inport  Port=5
  PP_CenterLineCalculat : Inport  Port=6
  TOS_VCAN_SignalVerification : Inport  Port=7
  LM_SignalVerification : Inport  Port=8
  PP_REElementType : Inport  Port=9
  Bus Creator : BusCreator  Inputs=9
  OFM_PortAdaptation : Subsystem
  Out1 : Outport
  wires:
  OFM_SignalVerification/1 -> OFM_PortAdaptation/1(OFMInfo)
  Bus Creator/1 -> Out1/1
  TOS_ProbInLaneCalculat/1 -> Bus Creator/5  "TOS_ProbInLaneCalculat"
  TLJ_TargetInLaneValidityJudg/1 -> Bus Creator/3  "TLJ_TargetInLaneValidityJudg"
  TOS_AddAttributes/1 -> Bus Creator/2  "TOS_AddAttributes"
  VIE_SignalVerification/1 -> Bus Creator/4  "VIE_SignalVerification"
  OFM_PortAdaptation/1(OFM_SignalVerification) -> Bus Creator/1  "OFM_SignalVerification"
  PP_CenterLineCalculat/1 -> Bus Creator/6  "PP_CenterLineCalculat"
  TOS_VCAN_SignalVerification/1 -> Bus Creator/7  "TOS_VCAN_SignalVerification"
  LM_SignalVerification/1 -> Bus Creator/8  "LM_SignalVerification"
  PP_REElementType/1 -> Bus Creator/9  "PP_REElementType"

== system PubIfDecisionTOS_MDL/TOS_20201112/TOS_2012080320/TOS/P0_Trajectory_V1.0 ==
  VehStandstill : Inport
  PsiDtOpt : Inport  Port=2
  VxvRef_ms : Inport  Port=3
  TOS_ACC_P0 : Inport  Port=4
  Bus Creator : BusCreator  Inputs=4
  Bus Creator1 : BusCreator  Inputs=4
  Bus Creator2 : BusCreator  Inputs=4
  Bus Creator3 : BusCreator  Inputs=7  OutDataTypeStr=Bus: TOS_P0_TARGET_LINE_BUS  NonVirtualBus=on
      settings: InheritFromInputs=off
  Bus Selector : BusSelector  OutputSignals=VehStandstill,PsiDtOpt,VxvRef_ms
  Bus Selector1 : BusSelector  OutputSignals=TOS_ACC_P0
  Bus Selector7 : BusSelector  OutputSignals=P0_EndPosition_dx,P0_EndPosition_dy
  Bus Selector8 : BusSelector  OutputSignals=P0_Counter
  Bus Selector9 : BusSelector  OutputSignals=VxvRef_ms
  CordinatConvert : Subsystem
  DataConfirm : Subsystem
  Terminator{,1..4} (5 alike) : Terminator
  TrackRecord : Subsystem
  TrgValidConfirm : Subsystem
  polyfit2 : MATLAB Function  TreatAsAtomicUnit=on
  TEM_P0_TARGET_LINE : Outport
  wires:
  TrackRecord/1(P0_TrackRecord) -> CordinatConvert/4(P0_TrackRecord_K1), [P0_TrackRecord], DataConfirm/1(P0_TrackRecord)  "P0_TrackRecord"
  TrgValidConfirm/1(P0_ID) -> Bus Creator/1
  TrgValidConfirm/4(P0_dy) -> Bus Creator/4
  TrgValidConfirm/3(P0_dx) -> Bus Creator/3
  TrgValidConfirm/2(P0_Counter) -> Bus Creator/2
  Bus Selector1/1 -> TrgValidConfirm/1(TOS_ACC_P0)  "<TOS_ACC_P0>"
  Bus Selector/3 -> CordinatConvert/3(VxvRef_ms)  "<VxvRef_ms>"
  Bus Selector/2 -> CordinatConvert/2(PsiDtOpt)  "<PsiDtOpt>"
  Bus Selector/1 -> CordinatConvert/1(VehStandstill)  "<VehStandstill>"
  Bus Creator2/1 -> Bus Selector1/1, Bus Selector/1, [P0_Trajectory_Sig]
  VehStandstill/1 -> Bus Creator2/1  "VehStandstill"
  PsiDtOpt/1 -> Bus Creator2/2  "PsiDtOpt"
  VxvRef_ms/1 -> Bus Creator2/3  "VxvRef_ms"
  Bus Creator1/1 -> TrackRecord/2(TrackRecord_CordinatConvert)  "TrackRecord_CordinatConvert"
  CordinatConvert/3(P0_Counter_TrackRecord_CordinatConvert_K1) -> Bus Creator1/3
  CordinatConvert/2(P0_dy_TrackRecord_CordinatConvert_K1) -> Bus Creator1/2
  CordinatConvert/1(P0_dx_TrackRecord_CordinatConvert_K1) -> Bus Creator1/1
  Bus Creator/1 -> [P0_TrgValidConfirm], TrackRecord/1(TOS_ACC_P0_Inf)  "TOS_ACC_P0_Inf"
  TOS_ACC_P0/1 -> Bus Creator2/4  "TOS_ACC_P0"
  CordinatConvert/4(P0_ID_TrackRecord_CordinatConvert_K1) -> Bus Creator1/4
  DataConfirm/1(dx) -> polyfit2/1("dx ")
  DataConfirm/2(dy) -> polyfit2/2("dy ")
  DataConfirm/3(P0_Counter) -> polyfit2/3("P0_Counter ")
  [P0_TrackRecord] -> Bus Selector7/1
  Bus Selector7/1 -> polyfit2/4(P0_EndPosition_dx)  "<P0_EndPosition_dx>"
  Bus Selector7/2 -> polyfit2/5(P0_EndPosition_dy)  "<P0_EndPosition_dy>"
  Bus Selector9/1 -> polyfit2/7(VxvRef_ms)  "<VxvRef_ms>"
  [P0_Trajectory_Sig] -> Bus Selector9/1
  Bus Selector8/1 -> polyfit2/6(P0_TrgValidConfirm_Counter)  "<P0_Counter>"
  [P0_TrgValidConfirm] -> Bus Selector8/1
  polyfit2/7(OTL_Cnt) -> Bus Creator3/7  "OTL_Cnt"
  polyfit2/6(OTL_Range) -> Bus Creator3/6  "OTL_Range"
  Bus Creator3/1 -> TEM_P0_TARGET_LINE/1
  polyfit2/4(OTL_C1) -> Bus Creator3/4  "OTL_C1"
  polyfit2/2(OTL_C3) -> Bus Creator3/2  "OTL_C3"
  polyfit2/3(OTL_C2) -> Bus Creator3/3  "OTL_C2"
  polyfit2/5(OTL_C0) -> Bus Creator3/5  "OTL_C0"
  polyfit2/1(OTL_Valid) -> Bus Creator3/1  "OTL_Valid"
  polyfit2/8(d_Start) -> Terminator/1  "TOS_P0_LINE_d_Start"
  polyfit2/9(d_End) -> Terminator1/1  "TOS_P0_LINE_d_End"
  polyfit2/11(dy) -> Terminator3/1
  polyfit2/10(P0_Counter) -> Terminator2/1
  polyfit2/12(dx) -> Terminator4/1

== system PubIfDecisionTOS_MDL/TOS_20201112/TOS_2012080320/PIL_1029/BoundaryCalculat/Lane_BoundaryCalculat ==
  OFM_SignalVerification : Inport
  TOS_AddAttributes : Inport  Port=2
  PP_CenterLineCalculat : Inport  Port=3
  Bus Creator1 : BusCreator  Inputs=3
  Bus Selector3 : BusSelector  OutputSignals=OFM_SignalVerification.TOS_OFMObjValid_Flag,OFM_SignalVerification.Object_Type,OFM_SignalVerification.Object_DX,OFM_SignalVerification.Object_MovingState,PP_CenterLineCalculat.TOS_PP_CurrentLaneWidth,PP_CenterLineCalculat.TOS_PP_LeftLaneWidth,PP_CenterLineCalculat.TOS_PP_RightLaneWidth
  Constant : Constant  Value=C_TOS_LaneLineCourseErrorFront  OutDataTypeStr=single
      settings: AttributesFormatString=P_TOS_LaneLineCourseError = 0.00014
  Constant1 : Constant  Value=C_TOS_LaneLineCourseErrorRear  OutDataTypeStr=single
      settings: AttributesFormatString=C_TOS_LaneLineCourseErrorRear = 0.00014
  Lane_Boundary : Subsystem
  SameLane_CoreArea_Boundary : Outport
  SameLane_EdgeLeft_Boundary : Outport  Port=2
  SameLane_EdgeRight_Boundary : Outport  Port=3
  LeftLane_CoreArea_Boundary : Outport  Port=4
  LeftLane_EdgeLeft_Boundary : Outport  Port=5
  LeftLane_EdgeRight_Boundary : Outport  Port=6
  RightLane_CoreArea_Boundary : Outport  Port=7
  RightLane_EdgeLeft_Boundary : Outport  Port=8
  RightLane_EdgeRight_Boundary : Outport  Port=9
  SameLane_BasicLaneWidth_ObserVale : Outport  Port=10
  LeftLane_BasicLaneWidth_ObserVale : Outport  Port=11
  RightLane_BasicLaneWidth_ObserVale : Outport  Port=12
  wires:
  Lane_Boundary/12(RightLane_BasicLaneWidth_ObserVale) -> RightLane_BasicLaneWidth_ObserVale/1
  Lane_Boundary/11(LeftLane_BasicLaneWidth_ObserVale) -> LeftLane_BasicLaneWidth_ObserVale/1
  Lane_Boundary/10(SameLane_BasicLaneWidth_ObserVale) -> SameLane_BasicLaneWidth_ObserVale/1
  Lane_Boundary/9(RightLane_EdgeRight_Boundary) -> RightLane_EdgeRight_Boundary/1
  Lane_Boundary/8(RightLane_EdgeLeft_Boundary) -> RightLane_EdgeLeft_Boundary/1
  Lane_Boundary/7(RightLane_CoreArea_Boundary) -> RightLane_CoreArea_Boundary/1
  Lane_Boundary/6(LeftLane_EdgeRight_Boundary) -> LeftLane_EdgeRight_Boundary/1
  Lane_Boundary/5(LeftLane_EdgeLeft_Boundary) -> LeftLane_EdgeLeft_Boundary/1
  Lane_Boundary/4(LeftLane_CoreArea_Boundary) -> LeftLane_CoreArea_Boundary/1
  Bus Selector3/3 -> Lane_Boundary/3(Object_DX)  "<Object_DX>"
  Constant1/1 -> Lane_Boundary/9(C_LaneLineCourseErrorRear)
  Bus Selector3/6 -> Lane_Boundary/6(PP_LeftLaneWidth)  "<TOS_PP_LeftLaneWidth>"
  Bus Selector3/2 -> Lane_Boundary/2(Object_Type)  "<Object_Type>"
  Bus Creator1/1 -> Bus Selector3/1
  Bus Selector3/4 -> Lane_Boundary/4(object_MovingState)  "<Object_MovingState>"
  Bus Selector3/1 -> Lane_Boundary/1(TOS_OFMObjValid_Flag)  "<TOS_OFMObjValid_Flag>"
  Bus Selector3/7 -> Lane_Boundary/7(PP_RightLaneWidth)  "<TOS_PP_RightLaneWidth>"
  Bus Selector3/5 -> Lane_Boundary/5(PP_CurrentLaneWidth)  "<TOS_PP_CurrentLaneWidth>"
  Constant/1 -> Lane_Boundary/8(C_LaneLineCourseErrorFront)
  Lane_Boundary/1(SameLane_CoreArea_Boundary) -> SameLane_CoreArea_Boundary/1
  Lane_Boundary/2(SameLane_EdgeLeft_Boundary) -> SameLane_EdgeLeft_Boundary/1
  Lane_Boundary/3(SameLane_EdgeRight_Boundary) -> SameLane_EdgeRight_Boundary/1
  PP_CenterLineCalculat/1 -> Bus Creator1/3  "PP_CenterLineCalculat"
  OFM_SignalVerification/1 -> Bus Creator1/1  "OFM_SignalVerification"
  TOS_AddAttributes/1 -> Bus Creator1/2  "TOS_AddAttributes"
